simulink model "DAQ_Write_Test"  (Simulink 4.00)
settings: Solver=FixedStepDiscrete  StartTime=0.0  StopTime=inf  FixedStep=0.05  RelTol=1e-3
libraries: DAQ_write_lib x1, simulink3 x1
settings Model: LastModifiedBy=bsaunder

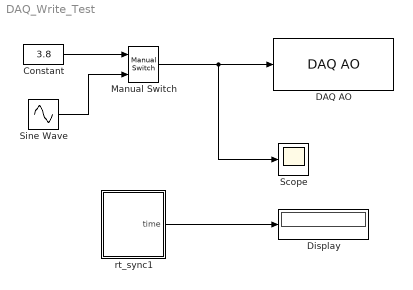
== system DAQ_Write_Test ==
  Constant : Constant  Value=3.8
  DAQ AO : DAQ_write_lib/DAQ AO  channel=1  Ts=0.05
  Display : Display
      settings: Format=short
  Manual Switch : simulink3/Nonlinear/Manual Switch  sw=0  action=0
  Scope : Scope
      settings: TimeRange=60  YMin=-5  YMax=5  SaveToWorkspace=off  SaveName=ScopeData  LimitDataPoints=on  MaxDataPoints=5000
  Sine Wave : Sin  SineType=Time-based  Amplitude=4  Bias=0  Frequency=0.1  Phase=0  Samples=10  SampleTime=0  Offset=0
  rt_sync1 : Subsystem  mask{Ts=0.05}
      mask prompts: Ts "Sample Time"
      settings: RTWFcnNameOpts=Auto  RTWFileNameOpts=Auto
      mask Display: fprintf('Real\n Time\n sync')
  wires:
  Sine Wave/1 -> Manual Switch/2
  Constant/1 -> Manual Switch/1
  Manual Switch/1 -> Scope/1, DAQ AO/1
  rt_sync1/1(time) -> Display/1

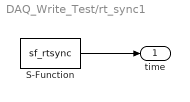
== system DAQ_Write_Test/rt_sync1 ==
  S-Function : S-Function  FunctionName=sf_rtsync  Parameters=Ts  PortCounts=[]  SFunctionModules=''
  time : Outport  Port=1
  wires:
  S-Function/1 -> time/1
